simulink model "sl_pursuit"  (R2017b)
settings: Solver=ode45  StartTime=0.0  StopTime=76  FixedStep=0.2  MaxStep=0.1  RelTol=1e-3  EnableMultiTasking=on
StopFcn:
  | set(0,'ShowHiddenHandles', 'on')
  | hold on
  | plot(robotpath(:,1), robotpath(:,2), 'r--', 'LineWidth', 2)
  | set(0,'ShowHiddenHandles', 'off')
undefined symbols (not defined in the file): numrows, robotpath, tseg
libraries: roblocks x2, simulink x1, simulink_need_slupdate x1
settings Model: Creator=pic  LastModifiedBy=ap
settings DataIOCC: SaveFormat=Array  SignalLoggingSaveFormat=ModelDataLogs  ReturnWorkspaceOutputs=on  TimeSaveName=t  OutputSaveName=y
settings OptimizationCC: ExpressionDepthLimit=2147483647  LifeSpan=inf
settings DebuggingCC: UnderspecifiedInitializationDetection=Classic  MergeDetectMultiDrivingBlocksExec=none  SolverPrmCheckMsg=warning  FcnCallInpInsideContextMsg=warning  AllowSymbolicDim=off  StateNameClashWarn=warning  SFUnexpectedBacktrackingDiag=warning  SFNoUnconditionalDefaultTransitionDiag=warning  SFExecutionAtInitializationDiag=none
settings HardwareCC: ProdBitPerPointer=32  ProdBitPerSizeT=32  ProdBitPerPtrDiffT=32  ProdLargestAtomicFloat=None  ProdIntDivRoundTo=Undefined  ProdEndianess=Unspecified  ProdWordSize=32  ProdHWDeviceType=32-bit Generic
settings ModelReferenceCC: PropagateSignalLabelsOutOfModel=off
settings CodeAppCC: StateflowObjectComments=on
settings GRTTargetCC: TargetLangStandard=C89/C90 (ANSI)  GeneratePreprocessorConditionals=Disable all  CombineOutputUpdateFcns=off  GRTInterface=on
settings ConfigComp: CovMetricSettings=dw  CovHtmlReporting=on  CovSaveCumulativeToWorkspaceVar=on  CovSaveSingleToWorkspaceVar=on  CovExternalEMLEnable=off

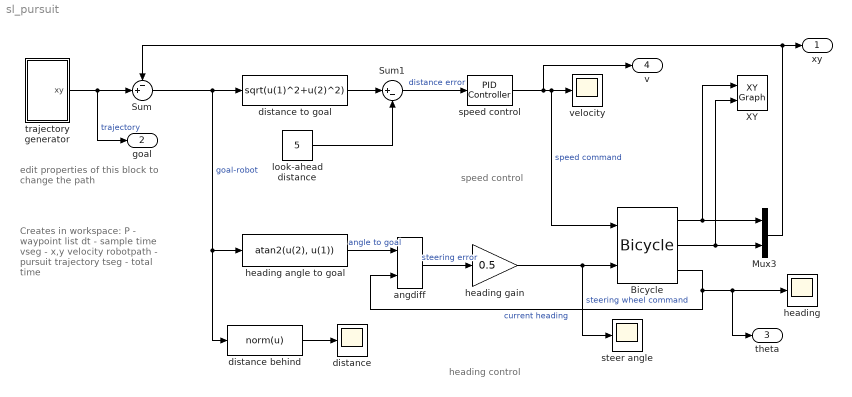
== system sl_pursuit ==
  note: speed control
  note: heading control
  note: Creates in workspace:
      | P - waypoint list
      | dt - sample time
      | vseg - x,y velocity
      | robotpath - pursuit trajectory
      | tseg - total time
  note: edit properties
      | of this block to
      | change the path
  Bicycle : roblocks/Vehicles/Bicycle  vlim=5  accel=1  alim=0.5  steer_rate=Inf  L=1  x0=[0, 0, 0]
  Mux3 : Mux  Inputs=2
  Sum : Sum  Inputs=-+|
  Sum1 : Sum  Inputs=|+-
  XY : simulink/Sinks/XY Graph  xmin=0  xmax=100  ymin=0  ymax=100  st=-1
  angdiff : roblocks/Toolbox/angdiff
  distance : Scope
  distance behind : MATLABFcn  MATLABFcn=norm(u)
  distance to goal : Fcn  Expr=sqrt(u(1)^2+u(2)^2)
  "heading " : Scope
  heading angle to goal : Fcn  Expr=atan2(u(2), u(1))
  heading gain : Gain  Gain=0.5
  look-ahead distance : Constant  Value=5
  speed control : simulink_need_slupdate/PID Controller  P=1  I=0.1  D=0
      settings: SourceProductName=Simulink
  steer angle : Scope
  trajectory generator : Subsystem  InitFcn=|
      | % create a path for the robot to follow
      | 
      | waypoints =[ 
      |   10 10
      |   10 60
      |   80 80
      |   50 10
      | ];
      | vseg = [2.5 2.5];
      | dt = 0.1;
      | robotpath = mstraj(waypoints(2:end,:), vseg, [], waypoints(1,:), dt, 0);
      | tseg = numrows(robotpath)*dt;
      | set_param('sl_pursuit', 'StopTime', num2str(sum(tseg)))
  velocity : Scope
  xy : Outport
  goal : Outport  Port=2
  theta : Outport  Port=3
  v : Outport  Port=4
  wires:
  Bicycle/1 -> Mux3/1, XY/1
  Bicycle/2 -> XY/2, Mux3/2
  Mux3/1 -> Sum/1, xy/1
  Sum/1 -> distance behind/1, heading angle to goal/1, distance to goal/1  "goal-robot"
  heading angle to goal/1 -> angdiff/1  "angle to goal"
  Bicycle/3 -> "heading "/1, theta/1, angdiff/2  "current heading"
  angdiff/1 -> heading gain/1  "steering error"
  heading gain/1 -> steer angle/1, Bicycle/2  "steering wheel command"
  speed control/1 -> Bicycle/1, velocity/1, v/1  "speed command"
  distance behind/1 -> distance/1
  trajectory generator/1(xy) -> goal/1, Sum/2  "trajectory"
  Sum1/1 -> speed control/1  "distance error"
  look-ahead distance/1 -> Sum1/2
  distance to goal/1 -> Sum1/1

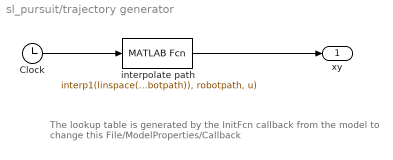
== system sl_pursuit/trajectory generator ==
  note: The lookup table is generated by the InitFcn callback from the model
      | to change this File/ModelProperties/Callback
  Clock : Clock
  interpolate path : MATLABFcn  MATLABFcn=interp1(linspace(0,tseg,numrows(robotpath)), robotpath, u)
  xy : Outport
  wires:
  Clock/1 -> interpolate path/1
  interpolate path/1 -> xy/1
